simulink model "current_model"  (R2023a)
settings: Solver=ode4  StartTime=0.0  StopTime=200  FixedStep=0.01  RelTol=1e-3
values from neighbouring files (symbols this model uses):
  max_current_direction_variation = 5.0    (= 5)    [init_current_model.m]
  max_current_speed_variation = 0.1    [init_current_model.m]
  mean_current_direction = 0.0    (= 0)    [init_current_model.m]
  mean_current_speed = 0.0    (= 0)    [init_current_model.m]
  time_constant_current_direction = 100.0    (= 100)    [init_current_model.m]
  time_constant_current_speed = 100.0    (= 100)    [init_current_model.m]
libraries: simulink x2, mssSimulink x1
settings Model: Creator=tobiasvt  LastModifiedBy=HalvorPlatou
settings SolverCC: AlgebraicLoopSolver=TrustRegion
settings DebuggingCC: UnconnectedInputMsg=warning  UnconnectedOutputMsg=warning  UnconnectedLineMsg=warning
settings ModelReferenceCC: EnableRefExpFcnMdlSchedulingChecks=on
settings SFSimCC: CustomCodeUndefinedFunction=UseInterfaceOnly
settings RTWCC: Description=FMU based on GRT (Functional Mock-up Unit)  SystemTargetFile=grtfmi.tlc  GenerateMakefile=off  TemplateMakefile=none  RetainRTWFile=on
settings STFCustomTargetCC: ConcurrentExecutionCompliant=off  CombineOutputUpdateFcns=on  GRTInterface=off  UseToolchainInfoCompliant=off  SystemTargetFile=grtfmi.tlc
settings GRTTargetCC: ParMdlRefBuildCompliant=off  CompOptLevelCompliant=off  ConcurrentExecutionCompliant=off  MatFileLogging=off  CPPClassGenCompliant=off  UseToolchainInfoCompliant=off

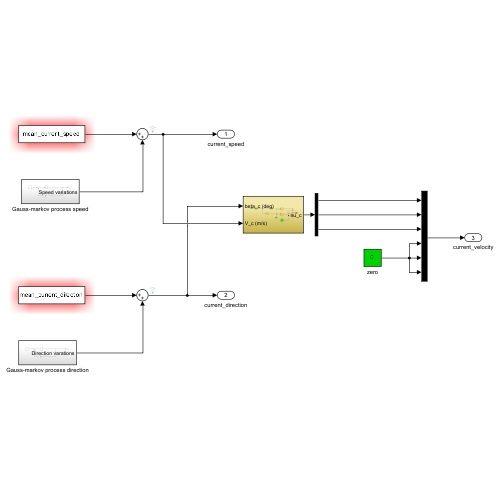
[thumbnail: Simulink's stored preview of the top-level diagram]
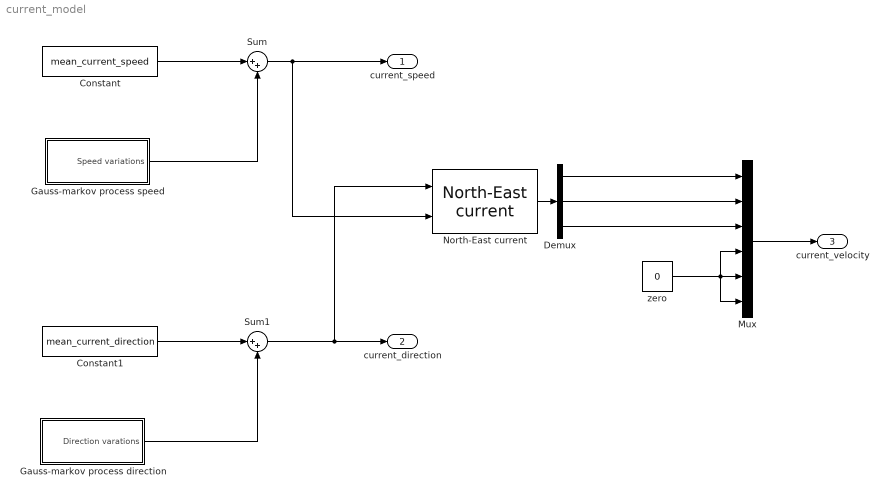
== system current_model ==
  Constant : Constant  Value=mean_current_speed
  Constant1 : Constant  Value=mean_current_direction
  Demux : Demux  Outputs=3
  Gauss-markov process direction : Subsystem
  Gauss-markov process speed : Subsystem
  Mux : Mux  Inputs=6
  North-East current : mssSimulink/Environment/Current/North-East current  SystemSampleTime=-1  VariantActivationTime=update diagram  Latency=0  AutoFrameSizeCalculation=off
  Sum : Sum  Inputs=|++
  Sum1 : Sum  Inputs=|++
  zero : Constant  Value=0
  current_speed : Outport  VectorParamsAs1DForOutWhenUnconnected=off
  current_direction : Outport  Port=2  VectorParamsAs1DForOutWhenUnconnected=off
  current_velocity : Outport  Port=3  VectorParamsAs1DForOutWhenUnconnected=off
  wires:
  Constant/1 -> Sum/1
  Gauss-markov process speed/1(Speed variations) -> Sum/2
  Gauss-markov process direction/1(Direction varations) -> Sum1/2
  Sum1/1 -> North-East current/1, current_direction/1
  Constant1/1 -> Sum1/1
  Sum/1 -> North-East current/2, current_speed/1
  North-East current/1 -> Demux/1
  Demux/1 -> Mux/1
  Demux/2 -> Mux/2
  Demux/3 -> Mux/3
  zero/1 -> Mux/4, Mux/6, Mux/5
  Mux/1 -> current_velocity/1

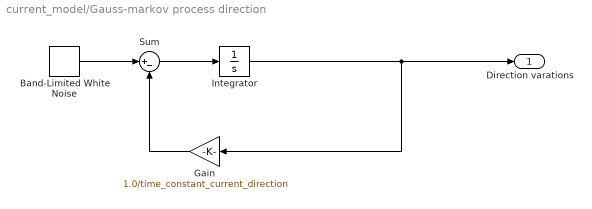
== system current_model/Gauss-markov process direction ==
  Band-Limited White Noise : simulink/Sources/Band-Limited White Noise  Cov=noise_power_current_direction  Ts=0.1  seed=321123
  Gain : Gain  Gain=1.0/time_constant_current_direction
  Integrator : Integrator  LimitOutput=on  UpperSaturationLimit=max_current_direction_variation  LowerSaturationLimit=-max_current_direction_variation
  Sum : Sum  Inputs=|+-
  Direction varations : Outport  VectorParamsAs1DForOutWhenUnconnected=off
  wires:
  Band-Limited White Noise/1 -> Sum/1
  Sum/1 -> Integrator/1
  Gain/1 -> Sum/2
  Integrator/1 -> Gain/1, Direction varations/1

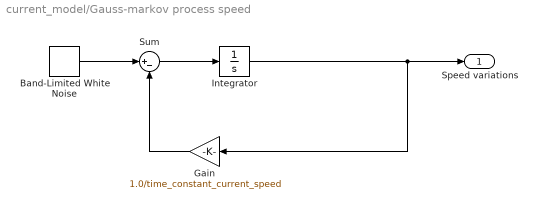
== system current_model/Gauss-markov process speed ==
  Band-Limited White Noise : simulink/Sources/Band-Limited White Noise  Cov=noise_power_current_speed  Ts=0.1  seed=123321
  Gain : Gain  Gain=1.0/time_constant_current_speed
  Integrator : Integrator  LimitOutput=on  UpperSaturationLimit=max_current_speed_variation  LowerSaturationLimit=-max_current_speed_variation
  Sum : Sum  Inputs=|+-
  Speed variations : Outport  VectorParamsAs1DForOutWhenUnconnected=off
  wires:
  Band-Limited White Noise/1 -> Sum/1
  Sum/1 -> Integrator/1
  Gain/1 -> Sum/2
  Integrator/1 -> Gain/1, Speed variations/1
